simulink model "test_sim"  (R2019a)
settings: Solver=VariableStepAuto  StartTime=0.0  StopTime=1  RelTol=1e-3
settings Model: Creator=Jan  LastModifiedBy=Jan

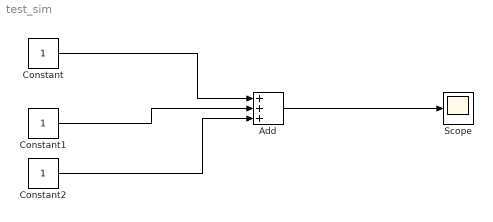
== system test_sim ==
  Add : Sum  Inputs=+++
  Constant : Constant
  Constant1 : Constant
  Constant2 : Constant
  Scope : Scope
  wires:
  Constant/1 -> Add/1
  Constant1/1 -> Add/2
  Add/1 -> Scope/1
  Constant2/1 -> Add/3
